simulink model "VehicleBackKin"  (R2024b)
settings: Solver=FixedStepAuto  StartTime=0.0  StopTime=inf  FixedStep=VehicleEnv.Ts  RelTol=1e-3
values from neighbouring files (symbols this model uses):
  em = ElectricMotor    [VehicleBackKinEnv.m]
  ess = VehicleEnv.ess    [VehicleBackKinEnv.m]
  fd = FinalDrive    [VehicleBackKinEnv.m]
  gb = Gearbox    [VehicleBackKinEnv.m]
  ice = Engine    [VehicleBackKinEnv.m]
  reward = VehicleEnv.reward    [VehicleBackKinEnv.m]
  selector_in = zeros(size(obs_info.Name))    [VehicleBackKinEnv.m]
  veh = Vehicle    [VehicleBackKinEnv.m]
  VehicleEnv = evalin("base","VehicleEnv")    [VehicleBackKinEnv.m]
  wh = Wheels    [VehicleBackKinEnv.m]
undefined symbols (not defined in the file or in its folder): agentSampleTime, cycle_insimulink, cycleTime, transfer_fun_coeff
libraries: simulink x3, rllib x1, autolibsharedcoreengin x1
(part 3 of 4)

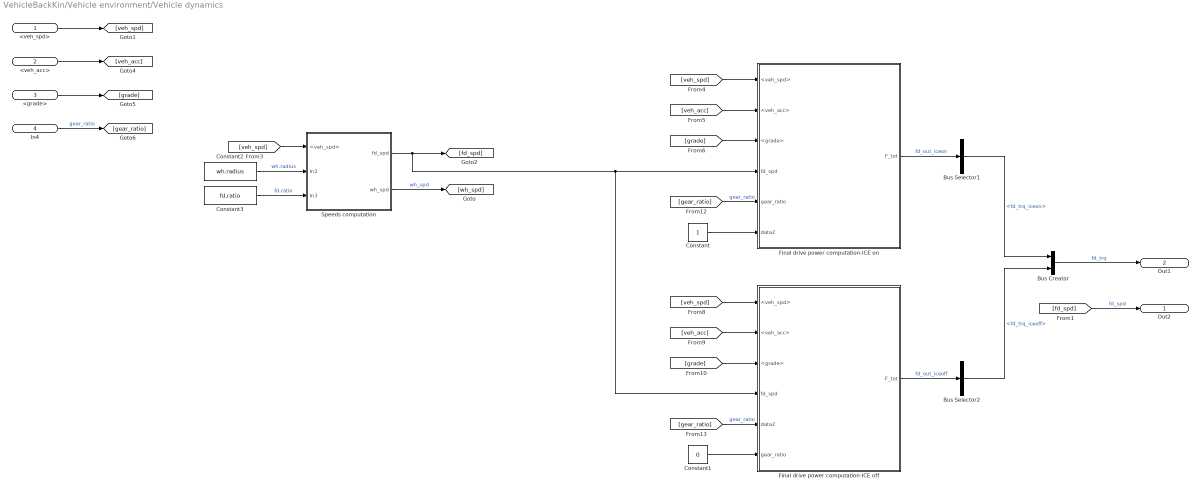
== system VehicleBackKin/Vehicle environment/Vehicle dynamics ==
  <veh_spd> : Inport
  <veh_acc> : Inport  Port=2
  <grade> : Inport  Port=3
  In4 : Inport  Port=4
  Bus Creator : BusCreator  Inputs=2
  Bus Selector1 : BusSelector  OutputSignals=fd_trq_iceon
  Bus Selector2 : BusSelector  OutputSignals=fd_trq_iceoff
  Constant : Constant
  Constant1 : Constant  Value=0
  Constant2 : Constant  Value=wh.radius
  Constant3 : Constant  Value=fd.ratio
  Final drive power computation-ICE off : Subsystem
  Final drive power computation-ICE on : Subsystem
  Speeds computation : Subsystem
  Out2 : Outport
  Out1 : Outport  Port=2
  wires:
  Speeds computation/1(fd_spd) -> [fd_spd], Final drive power computation-ICE off/4(fd_spd), Final drive power computation-ICE on/4(fd_spd)
  Speeds computation/2(wh_spd) -> [wh_spd]  "wh_spd"
  [fd_spd] -> Out2/1  "fd_spd"
  [gear_ratio] -> Final drive power computation-ICE on/5(gear_ratio)  "gear_ratio"
  <veh_spd>/1 -> [veh_spd]
  <veh_acc>/1 -> [veh_acc]
  <grade>/1 -> [grade]
  [veh_spd] -> Speeds computation/1(<veh_spd>)
  [veh_spd] -> Final drive power computation-ICE on/1(<veh_spd>)
  [veh_acc] -> Final drive power computation-ICE on/2(<veh_acc>)
  [grade] -> Final drive power computation-ICE on/3(<grade>)
  Constant/1 -> Final drive power computation-ICE on/6(data2)
  Constant1/1 -> Final drive power computation-ICE off/6(gear_ratio)
  [grade] -> Final drive power computation-ICE off/3(<grade>)
  [veh_spd] -> Final drive power computation-ICE off/1(<veh_spd>)
  [gear_ratio] -> Final drive power computation-ICE off/5(data2)  "gear_ratio"
  [veh_acc] -> Final drive power computation-ICE off/2(<veh_acc>)
  In4/1 -> [gear_ratio]  "gear_ratio"
  Constant2/1 -> Speeds computation/2(In2)  "wh.radius"
  Constant3/1 -> Speeds computation/3(In3)  "fd.ratio"
  Final drive power computation-ICE on/1(F_tot) -> Bus Selector1/1  "fd_out_iceon"
  Final drive power computation-ICE off/1(F_tot) -> Bus Selector2/1  "fd_out_iceoff"
  Bus Creator/1 -> Out1/1  "fd_trq"
  Bus Selector1/1 -> Bus Creator/1  "<fd_trq_iceon>"
  Bus Selector2/1 -> Bus Creator/2  "<fd_trq_iceoff>"

== system VehicleBackKin/Workspace saving/Testing ==
  In1 : Inport
  Bus Selector : BusSelector  OutputSignals=ice_out,batt_out,em_out,gb_out,veh_out,ems_out
  To Workspace1 : ToWorkspace  VariableName=ems_out  SaveFormat=Timeseries  SampleTime=-1
  To Workspace4 : ToWorkspace  VariableName=veh_out  SaveFormat=Timeseries  SampleTime=-1
  To Workspace5 : ToWorkspace  VariableName=gb_out  SaveFormat=Timeseries  SampleTime=-1
  To Workspace6 : ToWorkspace  VariableName=em_out  SaveFormat=Timeseries  SampleTime=-1
  To Workspace7 : ToWorkspace  VariableName=batt_out  SaveFormat=Timeseries  SampleTime=-1
  To Workspace8 : ToWorkspace  VariableName=ice_out  SaveFormat=Timeseries  SampleTime=-1
  wires:
  In1/1 -> Bus Selector/1
  Bus Selector/1 -> To Workspace8/1  "<ice_out>"
  Bus Selector/2 -> To Workspace7/1  "<batt_out>"
  Bus Selector/3 -> To Workspace6/1  "<em_out>"
  Bus Selector/4 -> To Workspace5/1  "<gb_out>"
  Bus Selector/5 -> To Workspace4/1  "<veh_out>"
  Bus Selector/6 -> To Workspace1/1  "<ems_out>"

== system VehicleBackKin/Workspace saving/Training ==
  In1 : Inport
  Bus Selector : BusSelector  OutputSignals=ice_out.ice_fuel_cum,batt_out.batt_soc
  To Workspace : ToWorkspace  VariableName=ice_fuel_cum  SaveFormat=Timeseries  SampleTime=1
  To Workspace1 : ToWorkspace  VariableName=batt_soc  SaveFormat=Timeseries  SampleTime=1
  wires:
  In1/1 -> Bus Selector/1
  Bus Selector/1 -> To Workspace/1  "<ice_fuel_cum>"
  Bus Selector/2 -> To Workspace1/1  "<batt_soc>"

== system VehicleBackKin/Reinforcement Learning controller/Reward/Dense ==
  note: Fuel penalty
  note: SoC penalty
  ice_fuel_rate : Inport
  agent_sample_time : Inport  Port=2
  batt_soc : Inport  Port=3
  Add : Sum  Inputs=+++
  Constant : Constant  Value=reward.soc_trg
  Constant1 : Constant  Value=reward.k1
  Gain : Gain  Gain=reward.k3
  Gain1 : Gain  Gain=reward.k2
  Product : Product
  SOC_reward_gain : Gain  Gain=reward.soc_gain
  Square : Math  Operator=square
  Subtract : Sum  Inputs=+-
  reward : Outport
  wires:
  Product/1 -> Gain1/1
  ice_fuel_rate/1 -> Product/1  "ice_fuel_rate"
  Add/1 -> reward/1  "reward"
  agent_sample_time/1 -> Product/2  "agent_sampleTime"
  Gain1/1 -> Add/2
  Constant1/1 -> Add/1
  Subtract/1 -> Square/1
  Constant/1 -> Subtract/2
  Gain/1 -> Add/3
  batt_soc/1 -> Subtract/1  "batt_soc"
  SOC_reward_gain/1 -> Gain/1
  Square/1 -> SOC_reward_gain/1

== system VehicleBackKin/Reinforcement Learning controller/Reward/Dense_multicycle ==
  note: Fuel penalty
  note: Distance percentage weigthing factor
  note: SoC penalty
  ice_fuel_rate : Inport
  agent_sample_time : Inport  Port=2
  batt_soc : Inport  Port=3
  veh_dist_tot : Inport  Port=4
  veh_dist_perc : Inport  Port=5
  Add : Sum  Inputs=+++
  Add1 : Sum
  Constant : Constant  Value=reward.soc_trg
  Constant1 : Constant  Value=reward.k1
  Divide : Product  Inputs=**/
  Divide1 : Product  Inputs=/*
  Gain : Gain  Gain=reward.k3*10
  Gain1 : Gain  Gain=reward.k2*10
  Gain2 : Gain  Gain=1/1000
  Product : Product
  Product1 : Product
  SOC_reward_gain : Gain  Gain=reward.soc_gain
  Square : Math  Operator=square
  Square1 : Math  Operator=square
  Subtract : Sum  Inputs=+-
  Subtract1 : Sum  Inputs=+-
  final_value : Constant
  initial_value : Constant  Value=0.3
  reward : Outport
  wires:
  Divide/1 -> Gain1/1
  ice_fuel_rate/1 -> Divide/1  "ice_fuel_rate"
  Add/1 -> reward/1  "reward"
  agent_sample_time/1 -> Divide/2  "agent_sampleTime"
  Gain1/1 -> Add/2
  Constant1/1 -> Add/1
  Constant/1 -> Subtract/2
  Gain/1 -> Add/3
  batt_soc/1 -> Subtract/1  "batt_soc"
  SOC_reward_gain/1 -> Gain/1
  veh_dist_tot/1 -> Gain2/1  "veh_dist_tot"
  Gain2/1 -> Divide1/1, Divide/3
  Subtract/1 -> Square/1
  Divide1/1 -> SOC_reward_gain/1
  Square/1 -> Product/1
  Product/1 -> Divide1/2
  Add1/1 -> Square1/1
  veh_dist_perc/1 -> Product1/1  "veh_dist_perc"
  Subtract1/1 -> Product1/2
  final_value/1 -> Subtract1/1
  Product1/1 -> Add1/1
  initial_value/1 -> Add1/2, Subtract1/2
  Square1/1 -> Product/2

== system VehicleBackKin/Reinforcement Learning controller/Reward/ECMS ==
  note: Fuel penalty
  note: Electric consumption penalty
  ice_fuel_rate : Inport
  batt_pwr : Inport  Port=2
  agent_sample_time : Inport  Port=3
  Add : Sum  Inputs=+++
  Constant1 : Constant  Value=reward.k1
  Equivalent fuel consumption : Subsystem
  Gain1 : Gain  Gain=reward.k2
  Product : Product
  reward : Outport
  wires:
  ice_fuel_rate/1 -> Product/1  "ice_fuel_rate"
  agent_sample_time/1 -> [Ts], Product/2  "agent_sampleTime"
  Product/1 -> Gain1/1
  Add/1 -> reward/1  "reward"
  Gain1/1 -> Add/2
  Constant1/1 -> Add/1
  batt_pwr/1 -> Equivalent fuel consumption/1(batt_pwr)  "batt_pwr"
  [Ts] -> Equivalent fuel consumption/2(In2)
  Equivalent fuel consumption/1(Out1) -> Add/3

== system VehicleBackKin/Reinforcement Learning controller/Reward/SOC_BC ==
  note: Fuel penalty
  note: SoC penalty
  ice_fuel_rate : Inport
  agent_sample_time : Inport  Port=2
  batt_soc : Inport  Port=3
  Add : Sum  Inputs=+++
  Constant1 : Constant  Value=reward.k1
  Gain1 : Gain  Gain=reward.k2
  Product : Product
  SoC boundary electric penalty : Subsystem
  reward : Outport
  wires:
  Constant1/1 -> Add/1
  Gain1/1 -> Add/2
  agent_sample_time/1 -> Product/2  "agent_sampleTime"
  Add/1 -> reward/1  "reward"
  ice_fuel_rate/1 -> Product/1  "ice_fuel_rate"
  Product/1 -> Gain1/1
  SoC boundary electric penalty/1(Out1) -> Add/3
  batt_soc/1 -> SoC boundary electric penalty/1(Input1)  "batt_soc"

== system VehicleBackKin/Reinforcement Learning controller/Reward/Sparse ==
  note: Fuel penalty
  note: Fuel penalty
  ice_fuel_rate : Inport
  batt_soc : Inport  Port=2
  is_done : Inport  Port=3
  agent_sample_time : Inport  Port=4
  Add : Sum  Inputs=+++
  Constant1 : Constant  Value=reward.k1
  Gain1 : Gain  Gain=reward.k2
  Product : Product
  SoC penalty : Subsystem  TreatAsAtomicUnit=on
  reward : Outport
  wires:
  SoC penalty/1(batt_soc_penalty) -> Add/2
  Add/1 -> reward/1
  is_done/1 -> SoC penalty/Enable  "is_done"
  agent_sample_time/1 -> Product/2  "agent_sampleTime"
  Product/1 -> Gain1/1
  ice_fuel_rate/1 -> Product/1  "ice_fuel_rate"
  Gain1/1 -> Add/3
  Constant1/1 -> Add/1
  batt_soc/1 -> SoC penalty/1(batt_soc)  "batt_soc"

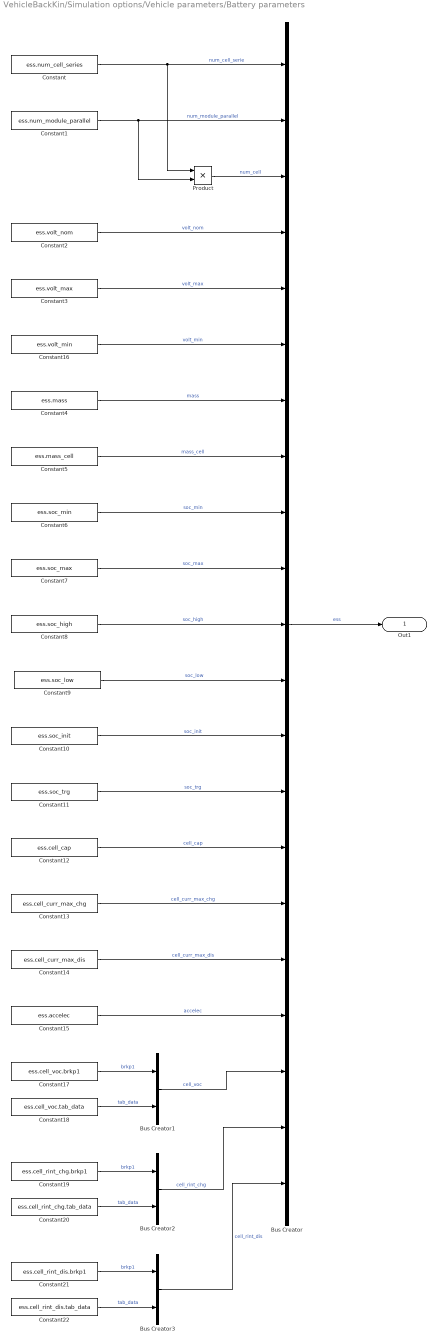
== system VehicleBackKin/Simulation options/Vehicle parameters/Battery parameters ==
  Bus Creator : BusCreator  Inputs=21
  Bus Creator1 : BusCreator  Inputs=2
  Bus Creator2 : BusCreator  Inputs=2
  Bus Creator3 : BusCreator  Inputs=2
  Constant : Constant  Value=ess.num_cell_series
  Constant1 : Constant  Value=ess.num_module_parallel
  Constant10 : Constant  Value=ess.soc_init
  Constant11 : Constant  Value=ess.soc_trg
  Constant12 : Constant  Value=ess.cell_cap
  Constant13 : Constant  Value=ess.cell_curr_max_chg
  Constant14 : Constant  Value=ess.cell_curr_max_dis
  Constant15 : Constant  Value=ess.accelec
  Constant16 : Constant  Value=ess.volt_min
  Constant17 : Constant  Value=ess.cell_voc.brkp1  VectorParams1D=off
  Constant18 : Constant  Value=ess.cell_voc.tab_data  VectorParams1D=off
  Constant19 : Constant  Value=ess.cell_rint_chg.brkp1  VectorParams1D=off
  Constant2 : Constant  Value=ess.volt_nom
  Constant20 : Constant  Value=ess.cell_rint_chg.tab_data  VectorParams1D=off
  Constant21 : Constant  Value=ess.cell_rint_dis.brkp1  VectorParams1D=off
  Constant22 : Constant  Value=ess.cell_rint_dis.tab_data  VectorParams1D=off
  Constant3 : Constant  Value=ess.volt_max
  Constant4 : Constant  Value=ess.mass
  Constant5 : Constant  Value=ess.mass_cell
  Constant6 : Constant  Value=ess.soc_min
  Constant7 : Constant  Value=ess.soc_max
  Constant8 : Constant  Value=ess.soc_high
  Constant9 : Constant  Value=ess.soc_low
  Product : Product
  Out1 : Outport
  wires:
  Constant/1 -> Bus Creator/1, Product/1  "num_cell_serie"
  Product/1 -> Bus Creator/3  "num_cell"
  Constant1/1 -> Bus Creator/2, Product/2  "num_module_parallel"
  Bus Creator/1 -> Out1/1  "ess"
  Constant2/1 -> Bus Creator/4  "volt_nom"
  Constant3/1 -> Bus Creator/5  "volt_max"
  Constant4/1 -> Bus Creator/7  "mass"
  Constant5/1 -> Bus Creator/8  "mass_cell"
  Constant6/1 -> Bus Creator/9  "soc_min"
  Constant7/1 -> Bus Creator/10  "soc_max"
  Constant8/1 -> Bus Creator/11  "soc_high"
  Constant14/1 -> Bus Creator/17  "cell_curr_max_dis"
  Constant15/1 -> Bus Creator/18  "accelec"
  Constant9/1 -> Bus Creator/12  "soc_low"
  Constant10/1 -> Bus Creator/13  "soc_init"
  Constant11/1 -> Bus Creator/14  "soc_trg"
  Constant12/1 -> Bus Creator/15  "cell_cap"
  Constant13/1 -> Bus Creator/16  "cell_curr_max_chg"
  Constant16/1 -> Bus Creator/6  "volt_min"
  Constant18/1 -> Bus Creator1/2  "tab_data"
  Constant17/1 -> Bus Creator1/1  "brkp1"
  Bus Creator1/1 -> Bus Creator/19  "cell_voc"
  Constant20/1 -> Bus Creator2/2  "tab_data"
  Constant19/1 -> Bus Creator2/1  "brkp1"
  Bus Creator2/1 -> Bus Creator/20  "cell_rint_chg"
  Constant22/1 -> Bus Creator3/2  "tab_data"
  Constant21/1 -> Bus Creator3/1  "brkp1"
  Bus Creator3/1 -> Bus Creator/21  "cell_rint_dis"

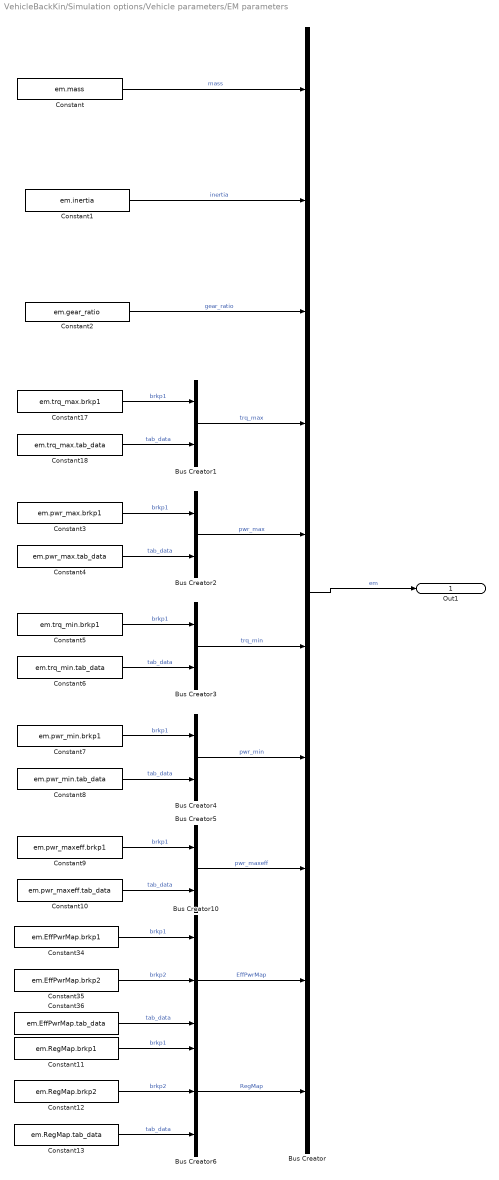
== system VehicleBackKin/Simulation options/Vehicle parameters/EM parameters ==
  Bus Creator : BusCreator  Inputs=10
  Bus Creator{1..5} (5 alike) : BusCreator  Inputs=2
  Bus Creator10 : BusCreator  Inputs=3
  Bus Creator6 : BusCreator  Inputs=3
  Constant : Constant  Value=em.mass
  Constant1 : Constant  Value=em.inertia
  Constant10 : Constant  Value=em.pwr_maxeff.tab_data  VectorParams1D=off
  Constant11 : Constant  Value=em.RegMap.brkp1  VectorParams1D=off
  Constant12 : Constant  Value=em.RegMap.brkp2  VectorParams1D=off
  Constant13 : Constant  Value=em.RegMap.tab_data  VectorParams1D=off
  Constant17 : Constant  Value=em.trq_max.brkp1  VectorParams1D=off
  Constant18 : Constant  Value=em.trq_max.tab_data  VectorParams1D=off
  Constant2 : Constant  Value=em.gear_ratio
  Constant3 : Constant  Value=em.pwr_max.brkp1  VectorParams1D=off
  Constant34 : Constant  Value=em.EffPwrMap.brkp1  VectorParams1D=off
  Constant35 : Constant  Value=em.EffPwrMap.brkp2  VectorParams1D=off
  Constant36 : Constant  Value=em.EffPwrMap.tab_data  VectorParams1D=off
  Constant4 : Constant  Value=em.pwr_max.tab_data  VectorParams1D=off
  Constant5 : Constant  Value=em.trq_min.brkp1  VectorParams1D=off
  Constant6 : Constant  Value=em.trq_min.tab_data  VectorParams1D=off
  Constant7 : Constant  Value=em.pwr_min.brkp1  VectorParams1D=off
  Constant8 : Constant  Value=em.pwr_min.tab_data  VectorParams1D=off
  Constant9 : Constant  Value=em.pwr_maxeff.brkp1  VectorParams1D=off
  Out1 : Outport
  wires:
  Bus Creator/1 -> Out1/1  "em"
  Constant1/1 -> Bus Creator/2  "inertia"
  Constant2/1 -> Bus Creator/3  "gear_ratio"
  Constant/1 -> Bus Creator/1  "mass"
  Constant17/1 -> Bus Creator1/1  "brkp1"
  Constant18/1 -> Bus Creator1/2  "tab_data"
  Bus Creator1/1 -> Bus Creator/4  "trq_max"
  Bus Creator2/1 -> Bus Creator/5  "pwr_max"
  Constant4/1 -> Bus Creator2/2  "tab_data"
  Constant3/1 -> Bus Creator2/1  "brkp1"
  Bus Creator3/1 -> Bus Creator/6  "trq_min"
  Constant6/1 -> Bus Creator3/2  "tab_data"
  Constant5/1 -> Bus Creator3/1  "brkp1"
  Bus Creator4/1 -> Bus Creator/7  "pwr_min"
  Constant8/1 -> Bus Creator4/2  "tab_data"
  Constant7/1 -> Bus Creator4/1  "brkp1"
  Bus Creator5/1 -> Bus Creator/8  "pwr_maxeff"
  Constant10/1 -> Bus Creator5/2  "tab_data"
  Constant9/1 -> Bus Creator5/1  "brkp1"
  Constant34/1 -> Bus Creator10/1  "brkp1"
  Constant35/1 -> Bus Creator10/2  "brkp2"
  Constant36/1 -> Bus Creator10/3  "tab_data"
  Bus Creator10/1 -> Bus Creator/9  "EffPwrMap"
  Bus Creator6/1 -> Bus Creator/10  "RegMap"
  Constant13/1 -> Bus Creator6/3  "tab_data"
  Constant12/1 -> Bus Creator6/2  "brkp2"
  Constant11/1 -> Bus Creator6/1  "brkp1"

== system VehicleBackKin/Simulation options/Vehicle parameters/Final drive parameters ==
  Bus Creator : BusCreator  Inputs=3
  Constant : Constant  Value=fd.ratio
  Constant1 : Constant  Value=fd.eff_max
  Constant2 : Constant  Value=fd.inertia
  Out1 : Outport
  wires:
  Constant2/1 -> Bus Creator/3  "inertia"
  Constant/1 -> Bus Creator/1  "ratio"
  Constant1/1 -> Bus Creator/2  "eff_max"
  Bus Creator/1 -> Out1/1  "fd"

== system VehicleBackKin/Simulation options/Vehicle parameters/Gearbox parameters ==
  Bus Creator : BusCreator  Inputs=6
  Constant : Constant  Value=gb.inertia_in
  Constant1 : Constant  Value=gb.inertia_out
  Constant2 : Constant  Value=gb.gear_idx
  Constant3 : Constant  Value=gb.gear_ratio
  EffTrqInMap : Subsystem
  EffTrqOutMap1 : Subsystem
  Out1 : Outport
  wires:
  Constant/1 -> Bus Creator/1  "inertia_in"
  Constant2/1 -> Bus Creator/3  "gear_idx"
  Constant1/1 -> Bus Creator/2  "inertia_out"
  Bus Creator/1 -> Out1/1  "gb"
  Constant3/1 -> Bus Creator/4  "gear_ratio"
  EffTrqInMap/1(Out1) -> Bus Creator/5
  EffTrqOutMap1/1(Out1) -> Bus Creator/6

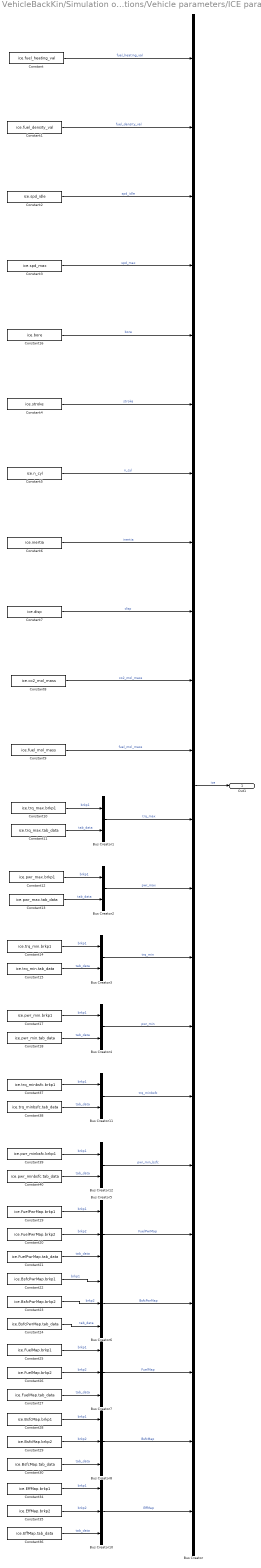
== system VehicleBackKin/Simulation options/Vehicle parameters/ICE parameters ==
  Bus Creator : BusCreator  Inputs=22
  Bus Creator{1..4,11..12} (6 alike) : BusCreator  Inputs=2
  Bus Creator{5..8,10} (5 alike) : BusCreator  Inputs=3
  Constant : Constant  Value=ice.fuel_heating_val
  Constant1 : Constant  Value=ice.fuel_density_val
  Constant10 : Constant  Value=ice.trq_max.brkp1  VectorParams1D=off
  Constant11 : Constant  Value=ice.trq_max.tab_data  VectorParams1D=off
  Constant12 : Constant  Value=ice.pwr_max.brkp1  VectorParams1D=off
  Constant13 : Constant  Value=ice.pwr_max.tab_data  VectorParams1D=off
  Constant14 : Constant  Value=ice.trq_min.brkp1  VectorParams1D=off
  Constant15 : Constant  Value=ice.trq_min.tab_data  VectorParams1D=off
  Constant16 : Constant  Value=ice.bore
  Constant17 : Constant  Value=ice.pwr_min.brkp1  VectorParams1D=off
  Constant18 : Constant  Value=ice.pwr_min.tab_data  VectorParams1D=off
  Constant19 : Constant  Value=ice.FuelPwrMap.brkp1  VectorParams1D=off
  Constant2 : Constant  Value=ice.spd_idle
  Constant20 : Constant  Value=ice.FuelPwrMap.brkp2  VectorParams1D=off
  Constant21 : Constant  Value=ice.FuelPwrMap.tab_data  VectorParams1D=off
  Constant22 : Constant  Value=ice.BsfcPwrMap.brkp1  VectorParams1D=off
  Constant23 : Constant  Value=ice.BsfcPwrMap.brkp2  VectorParams1D=off
  Constant24 : Constant  Value=ice.BsfcPwrMap.tab_data  VectorParams1D=off
  Constant25 : Constant  Value=ice.FuelMap.brkp1  VectorParams1D=off
  Constant26 : Constant  Value=ice.FuelMap.brkp2  VectorParams1D=off
  Constant27 : Constant  Value=ice.FuelMap.tab_data  VectorParams1D=off
  Constant28 : Constant  Value=ice.BsfcMap.brkp1  VectorParams1D=off
  Constant29 : Constant  Value=ice.BsfcMap.brkp2  VectorParams1D=off
  Constant3 : Constant  Value=ice.spd_max
  Constant30 : Constant  Value=ice.BsfcMap.tab_data  VectorParams1D=off
  Constant34 : Constant  Value=ice.EffMap.brkp1  VectorParams1D=off
  Constant35 : Constant  Value=ice.EffMap.brkp2  VectorParams1D=off
  Constant36 : Constant  Value=ice.EffMap.tab_data  VectorParams1D=off
  Constant37 : Constant  Value=ice.trq_minbsfc.brkp1  VectorParams1D=off
  Constant38 : Constant  Value=ice.trq_minbsfc.tab_data  VectorParams1D=off
  Constant39 : Constant  Value=ice.pwr_minbsfc.brkp1  VectorParams1D=off
  Constant4 : Constant  Value=ice.stroke
  Constant40 : Constant  Value=ice.pwr_minbsfc.tab_data  VectorParams1D=off
  Constant5 : Constant  Value=ice.n_cyl
  Constant6 : Constant  Value=ice.inertia
  Constant7 : Constant  Value=ice.disp
  Constant8 : Constant  Value=ice.co2_mol_mass
  Constant9 : Constant  Value=ice.fuel_mol_mass
  Out1 : Outport
  wires:
  Bus Creator/1 -> Out1/1  "ice"
  Constant1/1 -> Bus Creator/2  "fuel_density_val"
  Constant/1 -> Bus Creator/1  "fuel_heating_val"
  Constant2/1 -> Bus Creator/3  "spd_idle"
  Constant3/1 -> Bus Creator/4  "spd_max"
  Constant16/1 -> Bus Creator/5  "bore"
  Constant4/1 -> Bus Creator/6  "stroke"
  Constant5/1 -> Bus Creator/7  "n_cyl"
  Constant6/1 -> Bus Creator/8  "inertia"
  Constant7/1 -> Bus Creator/9  "disp"
  Constant8/1 -> Bus Creator/10  "co2_mol_mass"
  Constant9/1 -> Bus Creator/11  "fuel_mol_mass"
  Constant10/1 -> Bus Creator1/1  "brkp1"
  Constant11/1 -> Bus Creator1/2  "tab_data"
  Bus Creator1/1 -> Bus Creator/12  "trq_max"
  Bus Creator2/1 -> Bus Creator/13  "pwr_max"
  Constant13/1 -> Bus Creator2/2  "tab_data"
  Constant12/1 -> Bus Creator2/1  "brkp1"
  Constant14/1 -> Bus Creator3/1  "brkp1"
  Constant15/1 -> Bus Creator3/2  "tab_data"
  Constant18/1 -> Bus Creator4/2  "tab_data"
  Constant17/1 -> Bus Creator4/1  "brkp1"
  Constant19/1 -> Bus Creator5/1  "brkp1"
  Constant20/1 -> Bus Creator5/2  "brkp2"
  Constant21/1 -> Bus Creator5/3  "tab_data"
  Constant24/1 -> Bus Creator6/3  "tab_data"
  Constant23/1 -> Bus Creator6/2  "brkp2"
  Constant22/1 -> Bus Creator6/1  "brkp1"
  Constant25/1 -> Bus Creator7/1  "brkp1"
  Constant26/1 -> Bus Creator7/2  "brkp2"
  Constant27/1 -> Bus Creator7/3  "tab_data"
  Constant30/1 -> Bus Creator8/3  "tab_data"
  Bus Creator8/1 -> Bus Creator/21  "BsfcMap"
  Constant29/1 -> Bus Creator8/2  "brkp2"
  Constant28/1 -> Bus Creator8/1  "brkp1"
  Constant36/1 -> Bus Creator10/3  "tab_data"
  Bus Creator10/1 -> Bus Creator/22  "EffMap"
  Constant35/1 -> Bus Creator10/2  "brkp2"
  Constant34/1 -> Bus Creator10/1  "brkp1"
  Constant37/1 -> Bus Creator11/1  "brkp1"
  Constant38/1 -> Bus Creator11/2  "tab_data"
  Constant40/1 -> Bus Creator12/2  "tab_data"
  Constant39/1 -> Bus Creator12/1  "brkp1"
  Bus Creator7/1 -> Bus Creator/20  "FuelMap"
  Bus Creator6/1 -> Bus Creator/19  "BsfcPwrMap"
  Bus Creator5/1 -> Bus Creator/18  "FuelPwrMap"
  Bus Creator12/1 -> Bus Creator/17  "pwr_min_bsfc"
  Bus Creator11/1 -> Bus Creator/16  "trq_minbsfc"
  Bus Creator4/1 -> Bus Creator/15  "pwr_min"
  Bus Creator3/1 -> Bus Creator/14  "trq_min"

== system VehicleBackKin/Simulation options/Vehicle parameters/Vehicle paramateres ==
  Bus Creator : BusCreator  Inputs=6
  F0 : Constant  Value=veh.F0
  F1 : Constant  Value=veh.F1
  F2 : Constant  Value=veh.F2
  Subtract : Sum
  axal_base : Constant  Value=veh.axal_base
  body_mass : Constant  Value=veh.body_mass
  cargo_mass : Constant  Value=veh.cargo_mass
  cg_height : Constant  Value=veh.cg_height
  veh : Outport
  wires:
  Subtract/1 -> Bus Creator/3  "mass"
  cargo_mass/1 -> Subtract/1
  F0/1 -> Bus Creator/4  "F0"
  cg_height/1 -> Bus Creator/2  "cg_height"
  body_mass/1 -> Subtract/2
  F2/1 -> Bus Creator/6  "F2"
  F1/1 -> Bus Creator/5  "F1"
  axal_base/1 -> Bus Creator/1  "axal_base"
  Bus Creator/1 -> veh/1  "veh"

== system VehicleBackKin/Simulation options/Vehicle parameters/Wheels parameters ==
  Bus Creator : BusCreator  Inputs=3
  Constant : Constant  Value=wh.radius
  Constant1 : Constant  Value=wh.inertiaR
  Constant2 : Constant  Value=wh.inertiaF
  Out1 : Outport
  wires:
  Constant1/1 -> Bus Creator/2  "inertiaR"
  Constant/1 -> Bus Creator/1  "radius"
  Constant2/1 -> Bus Creator/3  "inertiaF"
  Bus Creator/1 -> Out1/1  "wh"

== system VehicleBackKin/Vehicle environment/Battery/Cell current calculation ==
  note: Cell parameters
  note: Current
  <cell_voc>1 : Inport
  In4 : Inport  Port=2
  Divide : Product  Inputs=*/
  Gain : Gain  Gain=4
  Gain1 : Gain  Gain=2
  Product : Product
  Square : Math  Operator=square
  Square Root : Sqrt
  Subtract : Sum  Inputs=+-
  Subtract1 : Sum  Inputs=+-
  Switch : Switch  SaturateOnIntegerOverflow=off  InputSameDT=off
  cell_init_chg : Lookup_n-D  NumberOfTableDimensions=1  BreakpointsForDimension1=ess.cell_rint_chg.brkp1  Table=ess.cell_rint_chg.tab_data  InternalRulePriority=Speed  RndMeth=Simplest
  cell_rint_dis : Lookup_n-D  NumberOfTableDimensions=1  BreakpointsForDimension1=ess.cell_rint_dis.brkp1  Table=ess.cell_rint_dis.tab_data  InternalRulePriority=Speed  RndMeth=Simplest
  cell_voc : Lookup_n-D  NumberOfTableDimensions=1  BreakpointsForDimension1=ess.cell_voc.brkp1  Table=ess.cell_voc.tab_data  InternalRulePriority=Speed  RndMeth=Simplest
  Out1 : Outport
  Out2 : Outport  Port=2
  Out3 : Outport  Port=3
  wires:
  cell_init_chg/1 -> Switch/3  "battc_Rchg"
  cell_voc/1 -> Out3/1, Subtract1/1, Square/1  "battc_voc"
  cell_rint_dis/1 -> Switch/1  "battc_Rdis"
  In4/1 -> [batt_soc]  "batt_soc"
  [battc_pwr] -> Switch/2
  <cell_voc>1/1 -> [battc_pwr]
  Switch/1 -> Gain1/1, Out2/1, Gain/1  "battc_R"
  Gain/1 -> Product/1
  [battc_pwr] -> Product/2
  Square/1 -> Subtract/1
  Product/1 -> Subtract/2
  Subtract/1 -> Square Root/1
  Square Root/1 -> Subtract1/2
  Subtract1/1 -> Divide/1
  Gain1/1 -> Divide/2
  Divide/1 -> Out1/1  "battc_curr"
  [batt_soc] -> cell_voc/1
  [batt_soc] -> cell_rint_dis/1
  [batt_soc] -> cell_init_chg/1

== system VehicleBackKin/Vehicle environment/Battery/Coulomb counting method ==
  note: State of charge
  note: Battery energy rate
  In1 : Inport
  <cell_cap> : Inport  Port=2
  Ah-->As : Gain  Gain=3600
  Divide : Product  Inputs=*/
  Gain : Gain  Gain=-1
  Gain1 : Gain  Gain=ess.volt_nom*ess.num_cell/1000
  Integrator : Integrator  InitialCondition=ess.soc_init
  Integrator1 : Integrator
  Product : Product
  Out1 : Outport
  Out2 : Outport  Port=2
  wires:
  Divide/1 -> Product/1, Gain/1
  Integrator/1 -> Out1/1  "batt_soc"
  In1/1 -> Divide/1  "battc_curr"
  <cell_cap>/1 -> Product/2, Ah-->As/1
  Ah-->As/1 -> Divide/2
  Gain/1 -> Integrator/1
  Product/1 -> Gain1/1
  Gain1/1 -> Integrator1/1
  Integrator1/1 -> Out2/1  "batt_en_rate [kWh]"

== system VehicleBackKin/Vehicle environment/ECU/Final drive torque management ==
  in_action : Inport
  In2 : Inport  Port=2
  In5 : Inport  Port=3
  <fd_trq_iceon> : Inport  Port=4
  <fd_trq_iceoff> : Inport  Port=5
  ice_state : Inport  Port=6
  Constant : Constant  Value=0
  Switch : Switch  Criteria=u2 > Threshold  SaturateOnIntegerOverflow=off  InputSameDT=off
  Switch1 : Switch  Criteria=u2 > Threshold  SaturateOnIntegerOverflow=off  InputSameDT=off
  Switch2 : Switch  Criteria=u2 > Threshold  SaturateOnIntegerOverflow=off  InputSameDT=off
  ice_pwr_dmd3 : Outport
  Out2 : Outport  Port=2
  Out1 : Outport  Port=3
  wires:
  ice_state/1 -> Switch/2, Switch2/2, Switch1/2
  <fd_trq_iceon>/1 -> Switch/1
  <fd_trq_iceoff>/1 -> Switch/3
  In2/1 -> Switch1/1
  In5/1 -> Switch1/3
  Switch/1 -> ice_pwr_dmd3/1  "fd_trq"
  Switch1/1 -> Out2/1  "fd_pwr"
  in_action/1 -> Switch2/1
  Constant/1 -> Switch2/3
  Switch2/1 -> Out1/1  "action"

== system VehicleBackKin/Vehicle environment/ECU/ICE state controller ==
  In1 : Inport
  Input2 : Inport  Port=2
  Constant : Constant
  Constant1 : Constant  Value=0
  Constant2 : Constant  Value=0
  Switch : Switch  Criteria=u2 > Threshold  Threshold=0.2  SaturateOnIntegerOverflow=off  InputSameDT=off
  Switch1 : Switch  Criteria=u2 > Threshold  SaturateOnIntegerOverflow=off  InputSameDT=off
  ice_pwr_dmd2 : Outport
  wires:
  Constant/1 -> Switch/1
  Constant1/1 -> Switch/3
  Switch/1 -> Switch1/1
  Input2/1 -> Switch/2
  In1/1 -> Switch1/2
  Constant2/1 -> Switch1/3
  Switch1/1 -> ice_pwr_dmd2/1  "ice_state"

== system VehicleBackKin/Vehicle environment/ECU/Limit computation ==
  In1 : Inport
  In2 : Inport  Port=2
  1-D Lookup Table : Lookup_n-D  NumberOfTableDimensions=1  BreakpointsForDimension1=ice.pwr_max.brkp1  Table=ice.pwr_max.tab_data  InternalRulePriority=Speed  RndMeth=Simplest
  1-D Lookup Table1 : Lookup_n-D  NumberOfTableDimensions=1  BreakpointsForDimension1=ice.pwr_min.brkp1  Table=ice.pwr_min.tab_data  InternalRulePriority=Speed  RndMeth=Simplest
  1-D Lookup Table2 : Lookup_n-D  NumberOfTableDimensions=1  BreakpointsForDimension1=ice.trq_max.brkp1  Table=ice.trq_max.tab_data  InternalRulePriority=Speed  RndMeth=Simplest
  1-D Lookup Table3 : Lookup_n-D  NumberOfTableDimensions=1  BreakpointsForDimension1=em.pwr_max.brkp1  Table=em.pwr_max.tab_data  InternalRulePriority=Speed  RndMeth=Simplest
  1-D Lookup Table4 : Lookup_n-D  NumberOfTableDimensions=1  BreakpointsForDimension1=em.pwr_min.brkp1  Table=em.pwr_min.tab_data  InternalRulePriority=Speed  RndMeth=Simplest
  ice_max_pwr : Outport
  ice_min_pwr : Outport  Port=2
  ice_max_trq : Outport  Port=3
  ice_max_pwr1 : Outport  Port=4
  ice_min_pwr1 : Outport  Port=5
  wires:
  In2/1 -> 1-D Lookup Table3/1, 1-D Lookup Table4/1
  1-D Lookup Table3/1 -> ice_max_pwr1/1  "em_pwr_max"
  In1/1 -> 1-D Lookup Table2/1, 1-D Lookup Table1/1, 1-D Lookup Table/1
  1-D Lookup Table2/1 -> ice_max_trq/1  "ice_trq_max"
  1-D Lookup Table4/1 -> ice_min_pwr1/1  "em_pwr_min"
  1-D Lookup Table/1 -> ice_max_pwr/1  "ice_pwr_max"
  1-D Lookup Table1/1 -> ice_min_pwr/1  "ice_pwr_min"

== system VehicleBackKin/Vehicle environment/ECU/Regenerative braking ==
  In1 : Inport
  In2 : Inport  Port=2
  Input : Inport  Port=3
  2-D Lookup Table : Lookup_n-D  BreakpointsForDimension1=em.RegMap.brkp2  BreakpointsForDimension2=em.RegMap.brkp1  Table=em.RegMap.tab_data  ExtrapMethod=Clip  InternalRulePriority=Speed  RndMeth=Simplest
      settings: InputPortMap=u0,u1
  Product2 : Product
  Scope : Scope
  Scope1 : Scope  NumInputPorts=2
  data2 : Outport
  wires:
  2-D Lookup Table/1 -> Scope/1, Product2/2  "reg_brk_factor"
  Product2/1 -> Scope1/2, data2/1  "em_pwr_reg"
  Input/1 -> Scope1/1, Product2/1
  In1/1 -> 2-D Lookup Table/1
  In2/1 -> 2-D Lookup Table/2

== system VehicleBackKin/Vehicle environment/ECU/Traction power demand ==
  ice_max_pwr : Inport
  ice_min_pwr : Inport  Port=2
  ice_max_trq : Inport  Port=3
  ice_max_pwr1 : Inport  Port=4
  ice_min_pwr1 : Inport  Port=5
  Input : Inport  Port=6
  In6 : Inport  Port=7
  ice_min_pwr2 : Inport  Port=8
  ice_max_trq1 : Inport  Port=9
  Constant : Constant  Value=0
  Product : Product
  Product1 : Product
  Saturation Dynamic : simulink/Discontinuities/Saturation Dynamic  OutMin=[]  OutMax=[]  OutDataTypeStr=Inherit: Same as second input  OutDataType=fixdt(1, 16)  OutScaling=2^-10  DoSatur=off
  Saturation Dynamic1 : simulink/Discontinuities/Saturation Dynamic  OutMin=[]  OutMax=[]  OutDataTypeStr=Inherit: Same as second input  OutDataType=fixdt(1, 16)  OutScaling=2^-10  DoSatur=off
  Subtract : Sum  Inputs=-+
  Switch : Switch  Criteria=u2 > Threshold  SaturateOnIntegerOverflow=off  InputSameDT=off
  ice_pwr_dmd : Outport
  Out2 : Outport  Port=2
  wires:
  Saturation Dynamic1/1 -> Out2/1  "em_pwr_trac"
  ice_min_pwr/1 -> Saturation Dynamic/3
  ice_min_pwr1/1 -> Saturation Dynamic1/3
  Product/1 -> Product1/1  "ice_trq"
  Switch/1 -> Subtract/1
  ice_max_pwr1/1 -> Saturation Dynamic1/1
  Subtract/1 -> Saturation Dynamic1/2  "em_pwr"
  ice_max_trq1/1 -> Product/1  "action"
  ice_max_pwr/1 -> Saturation Dynamic/1
  Saturation Dynamic/1 -> ice_pwr_dmd/1, Switch/1  "ice_pwr_trac"
  In6/1 -> Product1/2
  ice_min_pwr2/1 -> Switch/2
  Input/1 -> Subtract/2
  Product1/1 -> Saturation Dynamic/2  "ice_pwr"
  Constant/1 -> Switch/3
  ice_max_trq/1 -> Product/2

== system VehicleBackKin/Vehicle environment/Internal combustion engine/CO2 computation ==
  In3 : Inport
  <co2_mol_mass> : Inport  Port=2
  <fuel_mol_mass> : Inport  Port=3
  Divide : Product  Inputs=*/*
  Integrator : Integrator
  Out1 : Outport
  Out2 : Outport  Port=2
  wires:
  Divide/1 -> Integrator/1, Out1/1  "ice_co2_rate"
  In3/1 -> Divide/3
  <co2_mol_mass>/1 -> Divide/1
  <fuel_mol_mass>/1 -> Divide/2
  Integrator/1 -> Out2/1  "ice_co2_cum"

== system VehicleBackKin/Vehicle environment/Internal combustion engine/Fuel cut-off ==
  note: lessthan constant
  note: Cut-off
  In1 : Inport
  In2 : Inport  Port=2
  In3 : Inport  Port=3
  <spd_idle> : Inport  Port=4
  ice_pwr_dmd : Inport  Port=5
  AND : Logic  IconShape=distinctive  AllPortsSameDT=off  OutDataTypeStr=boolean
  Compare To Constant : simulink/Logic and Bit Operations/Compare To Constant  relop=<=  const=0  OutDataTypeStr=boolean
  Constant : Constant  Value=0
  Constant2 : Constant  Value=0  VectorParams1D=off  SampleTime=-1
  GreaterThan : RelationalOperator  Operator=>  OutDataTypeStr=boolean  RndMeth=Simplest  InputSameDT=off
  Switch : Switch  Criteria=u2 > Threshold  SaturateOnIntegerOverflow=off  InputSameDT=off
  Switch1 : Switch  Criteria=u2 > Threshold  SaturateOnIntegerOverflow=off  InputSameDT=off
  Out1 : Outport
  wires:
  <spd_idle>/1 -> GreaterThan/2
  In3/1 -> GreaterThan/1
  ice_pwr_dmd/1 -> Compare To Constant/1
  GreaterThan/1 -> AND/1
  Compare To Constant/1 -> AND/2
  Switch/1 -> Switch1/3
  AND/1 -> Switch1/2
  Switch1/1 -> Out1/1  "ice_fuel_rate"
  Constant/1 -> Switch/3
  In1/1 -> Switch/1  "ice_fuel_rate_map"
  In2/1 -> Switch/2  "ice_state"
  Constant2/1 -> Switch1/1

== system VehicleBackKin/Vehicle environment/Internal combustion engine/Speed calculation ==
  In1 : Inport
  ice_state : Inport  Port=2
  In2 : Inport  Port=3
  Constant : Constant  Value=0
  Max : MinMax  Function=max  Inputs=2
  Switch : Switch  Criteria=u2 > Threshold  SaturateOnIntegerOverflow=off  InputSameDT=off
  Out1 : Outport
  wires:
  Switch/1 -> Out1/1  "ice_spd"
  Constant/1 -> Switch/3
  In1/1 -> Max/1
  Max/1 -> Switch/1  "ice_spd"
  ice_state/1 -> Switch/2
  In2/1 -> Max/2

== system VehicleBackKin/Vehicle environment/Vehicle dynamics/Final drive power computation-ICE off ==
  <veh_spd> : Inport
  <veh_acc> : Inport  Port=2
  <grade> : Inport  Port=3
  fd_spd : Inport  Port=4
  data2 : Inport  Port=5
  gear_ratio : Inport  Port=6
  Road load power computation : Subsystem
  Vehicle equivalent mass : Subsystem
  F_tot : Outport
  wires:
  Vehicle equivalent mass/1(Out1) -> Road load power computation/5(In5)
  fd_spd/1 -> Road load power computation/4(fd_spd)
  <veh_acc>/1 -> Road load power computation/2(<veh_acc>)
  <veh_spd>/1 -> Road load power computation/1(<veh_spd>)
  gear_ratio/1 -> Vehicle equivalent mass/1(In2)
  <grade>/1 -> Road load power computation/3(<grade>)
  data2/1 -> Vehicle equivalent mass/2(data2)  "ice_state"
  Road load power computation/1(F_tot) -> F_tot/1

== system VehicleBackKin/Vehicle environment/Vehicle dynamics/Final drive power computation-ICE on ==
  <veh_spd> : Inport
  <veh_acc> : Inport  Port=2
  <grade> : Inport  Port=3
  fd_spd : Inport  Port=4
  gear_ratio : Inport  Port=5
  data2 : Inport  Port=6
  Road load power computation : Subsystem
  Vehicle equivalent mass : Subsystem
  F_tot : Outport
  wires:
  Vehicle equivalent mass/1(Out1) -> Road load power computation/5(In5)
  fd_spd/1 -> Road load power computation/4(fd_spd)
  <veh_acc>/1 -> Road load power computation/2(<veh_acc>)
  <veh_spd>/1 -> Road load power computation/1(<veh_spd>)
  gear_ratio/1 -> Vehicle equivalent mass/1(In2)
  <grade>/1 -> Road load power computation/3(<grade>)
  data2/1 -> Vehicle equivalent mass/2(data2)  "ice_state"
  Road load power computation/1(F_tot) -> F_tot/1

== system VehicleBackKin/Vehicle environment/Vehicle dynamics/Speeds computation ==
  <veh_spd> : Inport
  In2 : Inport  Port=2
  In3 : Inport  Port=3
  Divide : Product  Inputs=*/
  Product : Product
  fd_spd : Outport
  wh_spd : Outport  Port=2
  wires:
  Divide/1 -> wh_spd/1, Product/1  "wh_spd"
  <veh_spd>/1 -> Divide/1
  Product/1 -> fd_spd/1  "fd_spd"
  In3/1 -> Product/2
  In2/1 -> Divide/2

== system VehicleBackKin/Reinforcement Learning controller/Reward/ECMS/Equivalent fuel consumption ==
  batt_pwr : Inport
  In2 : Inport  Port=2
  Constant : Constant  Value=reward.eff_dis
  Constant2 : Constant  Value=reward.eff_chg
  Constant3 : Constant  Value=ice.fuel_heating_val
  Divide : Product  Inputs=*/
  Divide1 : Product  Inputs=*/
  Gain2 : Gain  Gain=reward.k3
  Product1 : Product
  Product2 : Product
  Switch : Switch  SaturateOnIntegerOverflow=off  InputSameDT=off
  Out1 : Outport
  wires:
  Product1/1 -> Switch/3
  Gain2/1 -> Divide1/1
  batt_pwr/1 -> Divide/1, Product1/1, Switch/2
  Constant/1 -> Divide/2
  In2/1 -> Product2/2  "Ts"
  Constant2/1 -> Product1/2
  Divide1/1 -> Product2/1
  Divide/1 -> Switch/1
  Constant3/1 -> Divide1/2
  Switch/1 -> Gain2/1
  Product2/1 -> Out1/1  "equivalent_fuel_consumption"

== system VehicleBackKin/Reinforcement Learning controller/Reward/SOC_BC/SoC boundary electric penalty ==
  Input1 : Inport
  Constant : Constant  Value=reward.soc_trg
  Constant1 : Constant  Value=reward.soc_trg
  Constant2 : Constant  Value=2*reward.soc_trg
  From Workspace : FromWorkspace  VariableName=reward_bc
  Gain : Gain  Gain=reward.k3
  Gain1 : Gain  Gain=reward.k3
  Gain2 : Gain  Gain=reward.soc_bc_gain
  GreaterThanOrEqual : RelationalOperator  OutDataTypeStr=boolean  RndMeth=Simplest  InputSameDT=off
  LowerThanOrEqua1 : RelationalOperator  Operator=<=  OutDataTypeStr=boolean  RndMeth=Simplest  InputSameDT=off
  OR : Logic  Operator=OR  IconShape=distinctive  AllPortsSameDT=off  OutDataTypeStr=boolean
  SOC_reward_gain : Gain  Gain=reward.soc_gain
  SOC_reward_gain1 : Gain  Gain=reward.soc_gain
  Square : Math  Operator=square
  Square1 : Math  Operator=square
  Subtract : Sum  Inputs=+-
  Subtract1 : Sum  Inputs=+-
  Subtract2 : Sum  Inputs=-+
  Switch : Switch  Criteria=u2 > Threshold  SaturateOnIntegerOverflow=off  InputSameDT=off
  Out1 : Outport
  wires:
  From Workspace/1 -> Subtract2/1, GreaterThanOrEqual/2  "soc_bc_up"
  Gain1/1 -> Gain2/1
  Subtract2/1 -> LowerThanOrEqua1/2  "soc_bc_low"
  OR/1 -> Switch/2
  Constant2/1 -> Subtract2/2
  GreaterThanOrEqual/1 -> OR/1
  Gain/1 -> Switch/1
  LowerThanOrEqua1/1 -> OR/2
  [batt_soc] -> LowerThanOrEqua1/1
  Switch/1 -> Out1/1  "batt_soc_penalty"
  Input1/1 -> [batt_soc]
  Constant/1 -> Subtract/2
  Square/1 -> SOC_reward_gain/1
  SOC_reward_gain/1 -> Gain/1
  [batt_soc] -> Subtract/1  "batt_soc"
  Subtract/1 -> Square/1
  [batt_soc] -> GreaterThanOrEqual/1
  SOC_reward_gain1/1 -> Gain1/1
  Subtract1/1 -> Square1/1
  Constant1/1 -> Subtract1/2
  [batt_soc] -> Subtract1/1  "batt_soc"
  Square1/1 -> SOC_reward_gain1/1
  Gain2/1 -> Switch/3

== system VehicleBackKin/Reinforcement Learning controller/Reward/Sparse/SoC penalty ==
  batt_soc : Inport
  Enable : EnablePort  StatesWhenEnabling=reset
  Constant3 : Constant  Value=reward.soc_trg
  Gain : Gain  Gain=reward.k3
  SOC_reward_gain : Gain  Gain=reward.soc_gain
  Square : Math  Operator=square
  Subtract1 : Sum  Inputs=+-
  batt_soc_penalty : Outport
  wires:
  Constant3/1 -> Subtract1/2
  Subtract1/1 -> Square/1
  batt_soc/1 -> Subtract1/1  "batt_soc"
  SOC_reward_gain/1 -> Gain/1
  Square/1 -> SOC_reward_gain/1
  Gain/1 -> batt_soc_penalty/1  "batt_soc_penalty"

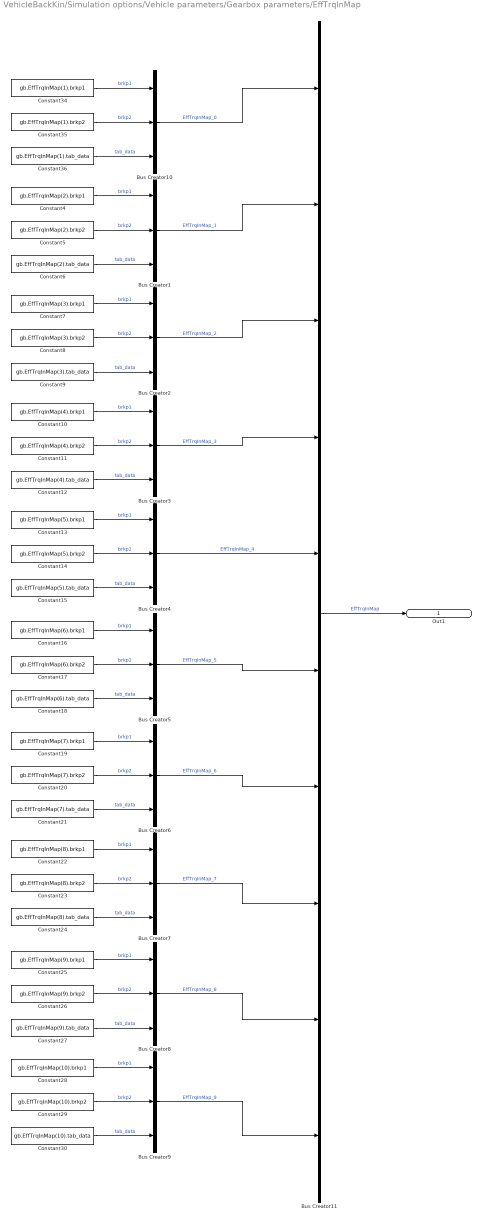
== system VehicleBackKin/Simulation options/Vehicle parameters/Gearbox parameters/EffTrqInMap ==
  Bus Creator{1..10} (10 alike) : BusCreator  Inputs=3
  Bus Creator11 : BusCreator  Inputs=10
  Constant10 : Constant  Value=gb.EffTrqInMap(4).brkp1
  Constant11 : Constant  Value=gb.EffTrqInMap(4).brkp2
  Constant12 : Constant  Value=gb.EffTrqInMap(4).tab_data
  Constant13 : Constant  Value=gb.EffTrqInMap(5).brkp1
  Constant14 : Constant  Value=gb.EffTrqInMap(5).brkp2
  Constant15 : Constant  Value=gb.EffTrqInMap(5).tab_data
  Constant16 : Constant  Value=gb.EffTrqInMap(6).brkp1
  Constant17 : Constant  Value=gb.EffTrqInMap(6).brkp2
  Constant18 : Constant  Value=gb.EffTrqInMap(6).tab_data
  Constant19 : Constant  Value=gb.EffTrqInMap(7).brkp1
  Constant20 : Constant  Value=gb.EffTrqInMap(7).brkp2
  Constant21 : Constant  Value=gb.EffTrqInMap(7).tab_data
  Constant22 : Constant  Value=gb.EffTrqInMap(8).brkp1
  Constant23 : Constant  Value=gb.EffTrqInMap(8).brkp2
  Constant24 : Constant  Value=gb.EffTrqInMap(8).tab_data
  Constant25 : Constant  Value=gb.EffTrqInMap(9).brkp1
  Constant26 : Constant  Value=gb.EffTrqInMap(9).brkp2
  Constant27 : Constant  Value=gb.EffTrqInMap(9).tab_data
  Constant28 : Constant  Value=gb.EffTrqInMap(10).brkp1
  Constant29 : Constant  Value=gb.EffTrqInMap(10).brkp2
  Constant30 : Constant  Value=gb.EffTrqInMap(10).tab_data
  Constant34 : Constant  Value=gb.EffTrqInMap(1).brkp1
  Constant35 : Constant  Value=gb.EffTrqInMap(1).brkp2
  Constant36 : Constant  Value=gb.EffTrqInMap(1).tab_data
  Constant4 : Constant  Value=gb.EffTrqInMap(2).brkp1
  Constant5 : Constant  Value=gb.EffTrqInMap(2).brkp2
  Constant6 : Constant  Value=gb.EffTrqInMap(2).tab_data
  Constant7 : Constant  Value=gb.EffTrqInMap(3).brkp1
  Constant8 : Constant  Value=gb.EffTrqInMap(3).brkp2
  Constant9 : Constant  Value=gb.EffTrqInMap(3).tab_data
  Out1 : Outport
  wires:
  Constant18/1 -> Bus Creator5/3  "tab_data"
  Constant22/1 -> Bus Creator7/1  "brkp1"
  Bus Creator3/1 -> Bus Creator11/4  "EffTrqInMap_3"
  Constant29/1 -> Bus Creator9/2  "brkp2"
  Constant7/1 -> Bus Creator2/1  "brkp1"
  Constant5/1 -> Bus Creator1/2  "brkp2"
  Constant10/1 -> Bus Creator3/1  "brkp1"
  Constant25/1 -> Bus Creator8/1  "brkp1"
  Constant19/1 -> Bus Creator6/1  "brkp1"
  Constant35/1 -> Bus Creator10/2  "brkp2"
  Bus Creator1/1 -> Bus Creator11/2  "EffTrqInMap_1"
  Bus Creator5/1 -> Bus Creator11/6  "EffTrqInMap_5"
  Constant11/1 -> Bus Creator3/2  "brkp2"
  Constant12/1 -> Bus Creator3/3  "tab_data"
  Bus Creator8/1 -> Bus Creator11/9  "EffTrqInMap_8"
  Constant4/1 -> Bus Creator1/1  "brkp1"
  Constant17/1 -> Bus Creator5/2  "brkp2"
  Constant21/1 -> Bus Creator6/3  "tab_data"
  Bus Creator7/1 -> Bus Creator11/8  "EffTrqInMap_7"
  Constant16/1 -> Bus Creator5/1  "brkp1"
  Constant36/1 -> Bus Creator10/3  "tab_data"
  Constant24/1 -> Bus Creator7/3  "tab_data"
  Constant34/1 -> Bus Creator10/1  "brkp1"
  Constant28/1 -> Bus Creator9/1  "brkp1"
  Bus Creator10/1 -> Bus Creator11/1  "EffTrqInMap_0"
  Constant30/1 -> Bus Creator9/3  "tab_data"
  Constant23/1 -> Bus Creator7/2  "brkp2"
  Bus Creator11/1 -> Out1/1  "EffTrqInMap"
  Constant20/1 -> Bus Creator6/2  "brkp2"
  Constant26/1 -> Bus Creator8/2  "brkp2"
  Constant13/1 -> Bus Creator4/1  "brkp1"
  Constant14/1 -> Bus Creator4/2  "brkp2"
  Constant15/1 -> Bus Creator4/3  "tab_data"
  Bus Creator2/1 -> Bus Creator11/3  "EffTrqInMap_2"
  Bus Creator9/1 -> Bus Creator11/10  "EffTrqInMap_9"
  Bus Creator4/1 -> Bus Creator11/5  "EffTrqInMap_4"
  Constant9/1 -> Bus Creator2/3  "tab_data"
  Constant27/1 -> Bus Creator8/3  "tab_data"
  Constant8/1 -> Bus Creator2/2  "brkp2"
  Bus Creator6/1 -> Bus Creator11/7  "EffTrqInMap_6"
  Constant6/1 -> Bus Creator1/3  "tab_data"

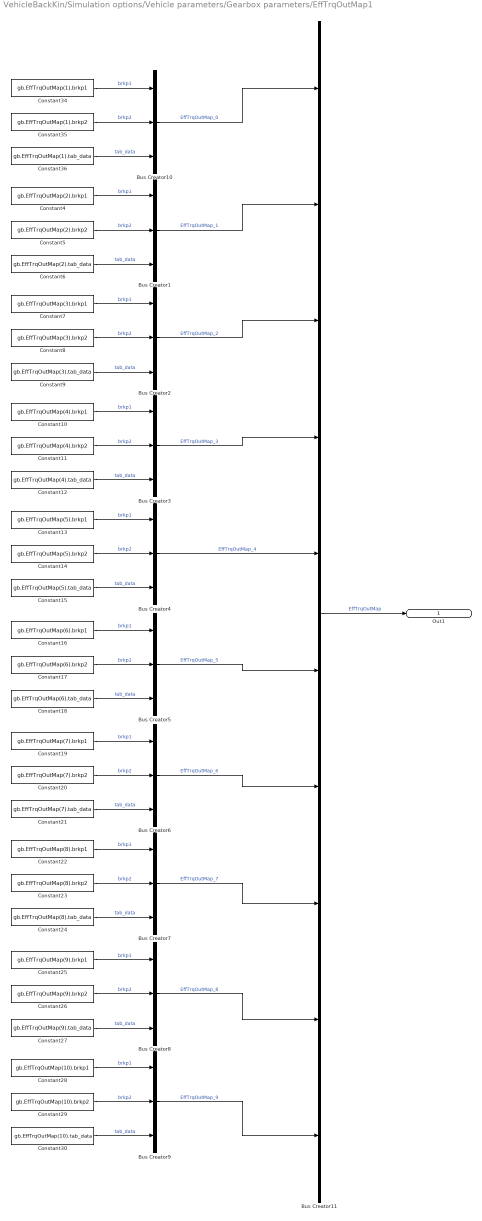
== system VehicleBackKin/Simulation options/Vehicle parameters/Gearbox parameters/EffTrqOutMap1 ==
  Bus Creator{1..10} (10 alike) : BusCreator  Inputs=3
  Bus Creator11 : BusCreator  Inputs=10
  Constant10 : Constant  Value=gb.EffTrqOutMap(4).brkp1
  Constant11 : Constant  Value=gb.EffTrqOutMap(4).brkp2
  Constant12 : Constant  Value=gb.EffTrqOutMap(4).tab_data
  Constant13 : Constant  Value=gb.EffTrqOutMap(5).brkp1
  Constant14 : Constant  Value=gb.EffTrqOutMap(5).brkp2
  Constant15 : Constant  Value=gb.EffTrqOutMap(5).tab_data
  Constant16 : Constant  Value=gb.EffTrqOutMap(6).brkp1
  Constant17 : Constant  Value=gb.EffTrqOutMap(6).brkp2
  Constant18 : Constant  Value=gb.EffTrqOutMap(6).tab_data
  Constant19 : Constant  Value=gb.EffTrqOutMap(7).brkp1
  Constant20 : Constant  Value=gb.EffTrqOutMap(7).brkp2
  Constant21 : Constant  Value=gb.EffTrqOutMap(7).tab_data
  Constant22 : Constant  Value=gb.EffTrqOutMap(8).brkp1
  Constant23 : Constant  Value=gb.EffTrqOutMap(8).brkp2
  Constant24 : Constant  Value=gb.EffTrqOutMap(8).tab_data
  Constant25 : Constant  Value=gb.EffTrqOutMap(9).brkp1
  Constant26 : Constant  Value=gb.EffTrqOutMap(9).brkp2
  Constant27 : Constant  Value=gb.EffTrqOutMap(9).tab_data
  Constant28 : Constant  Value=gb.EffTrqOutMap(10).brkp1
  Constant29 : Constant  Value=gb.EffTrqOutMap(10).brkp2
  Constant30 : Constant  Value=gb.EffTrqOutMap(10).tab_data
  Constant34 : Constant  Value=gb.EffTrqOutMap(1).brkp1
  Constant35 : Constant  Value=gb.EffTrqOutMap(1).brkp2
  Constant36 : Constant  Value=gb.EffTrqOutMap(1).tab_data
  Constant4 : Constant  Value=gb.EffTrqOutMap(2).brkp1
  Constant5 : Constant  Value=gb.EffTrqOutMap(2).brkp2
  Constant6 : Constant  Value=gb.EffTrqOutMap(2).tab_data
  Constant7 : Constant  Value=gb.EffTrqOutMap(3).brkp1
  Constant8 : Constant  Value=gb.EffTrqOutMap(3).brkp2
  Constant9 : Constant  Value=gb.EffTrqOutMap(3).tab_data
  Out1 : Outport
  wires:
  Constant18/1 -> Bus Creator5/3  "tab_data"
  Constant22/1 -> Bus Creator7/1  "brkp1"
  Bus Creator3/1 -> Bus Creator11/4  "EffTrqOutMap_3"
  Constant29/1 -> Bus Creator9/2  "brkp2"
  Constant7/1 -> Bus Creator2/1  "brkp1"
  Constant5/1 -> Bus Creator1/2  "brkp2"
  Constant10/1 -> Bus Creator3/1  "brkp1"
  Constant25/1 -> Bus Creator8/1  "brkp1"
  Constant19/1 -> Bus Creator6/1  "brkp1"
  Constant35/1 -> Bus Creator10/2  "brkp2"
  Bus Creator1/1 -> Bus Creator11/2  "EffTrqOutMap_1"
  Bus Creator5/1 -> Bus Creator11/6  "EffTrqOutMap_5"
  Constant11/1 -> Bus Creator3/2  "brkp2"
  Constant12/1 -> Bus Creator3/3  "tab_data"
  Bus Creator8/1 -> Bus Creator11/9  "EffTrqOutMap_8"
  Constant4/1 -> Bus Creator1/1  "brkp1"
  Constant17/1 -> Bus Creator5/2  "brkp2"
  Constant21/1 -> Bus Creator6/3  "tab_data"
  Bus Creator7/1 -> Bus Creator11/8  "EffTrqOutMap_7"
  Constant16/1 -> Bus Creator5/1  "brkp1"
  Constant36/1 -> Bus Creator10/3  "tab_data"
  Constant24/1 -> Bus Creator7/3  "tab_data"
  Constant34/1 -> Bus Creator10/1  "brkp1"
  Constant28/1 -> Bus Creator9/1  "brkp1"
  Bus Creator10/1 -> Bus Creator11/1  "EffTrqOutMap_0"
  Constant30/1 -> Bus Creator9/3  "tab_data"
  Constant23/1 -> Bus Creator7/2  "brkp2"
  Bus Creator11/1 -> Out1/1  "EffTrqOutMap"
  Constant20/1 -> Bus Creator6/2  "brkp2"
  Constant26/1 -> Bus Creator8/2  "brkp2"
  Constant13/1 -> Bus Creator4/1  "brkp1"
  Constant14/1 -> Bus Creator4/2  "brkp2"
  Constant15/1 -> Bus Creator4/3  "tab_data"
  Bus Creator2/1 -> Bus Creator11/3  "EffTrqOutMap_2"
  Bus Creator9/1 -> Bus Creator11/10  "EffTrqOutMap_9"
  Bus Creator4/1 -> Bus Creator11/5  "EffTrqOutMap_4"
  Constant9/1 -> Bus Creator2/3  "tab_data"
  Constant27/1 -> Bus Creator8/3  "tab_data"
  Constant8/1 -> Bus Creator2/2  "brkp2"
  Bus Creator6/1 -> Bus Creator11/7  "EffTrqOutMap_6"
  Constant6/1 -> Bus Creator1/3  "tab_data"

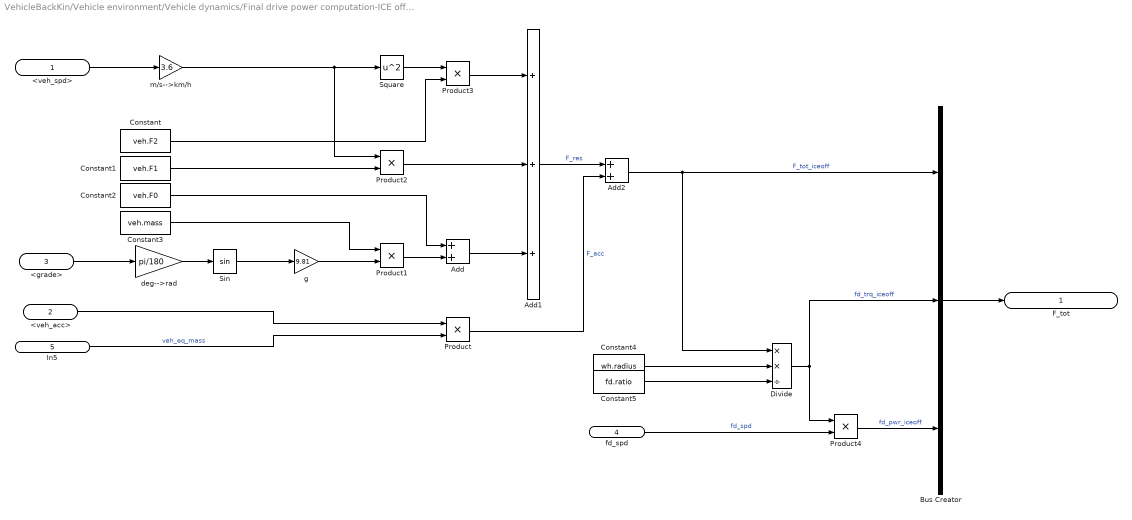
== system VehicleBackKin/Vehicle environment/Vehicle dynamics/Final drive power computation-ICE off/Road load power computation ==
  <veh_spd> : Inport
  <veh_acc> : Inport  Port=2
  <grade> : Inport  Port=3
  fd_spd : Inport  Port=4
  In5 : Inport  Port=5
  Add : Sum
  Add1 : Sum  Inputs=+++
  Add2 : Sum
  Bus Creator : BusCreator  Inputs=3
  Constant : Constant  Value=veh.F2
  Constant1 : Constant  Value=veh.F1
  Constant2 : Constant  Value=veh.F0
  Constant3 : Constant  Value=veh.mass
  Constant4 : Constant  Value=wh.radius
  Constant5 : Constant  Value=fd.ratio
  Divide : Product  Inputs=**/
  Product{,1..4} (5 alike) : Product
  Sin : Trigonometry
  Square : Math  Operator=square
  deg-->rad : Gain  Gain=pi/180
  g : Gain  Gain=9.81
  m/s-->km/h : Gain  Gain=3.6
  F_tot : Outport
  wires:
  <veh_spd>/1 -> m/s-->km/h/1
  <grade>/1 -> deg-->rad/1
  deg-->rad/1 -> Sin/1
  Constant1/1 -> Product2/2
  Sin/1 -> g/1
  m/s-->km/h/1 -> Product2/1, Square/1
  Constant2/1 -> Add/1
  Constant3/1 -> Product1/1
  g/1 -> Product1/2
  Product2/1 -> Add1/2
  Product1/1 -> Add/2
  Product3/1 -> Add1/1
  Add1/1 -> Add2/1  "F_res"
  Add/1 -> Add1/3
  <veh_acc>/1 -> Product/1
  In5/1 -> Product/2  "veh_eq_mass"
  Add2/1 -> Divide/1, Bus Creator/1  "F_tot_iceoff"
  Product/1 -> Add2/2  "F_acc"
  Constant/1 -> Product3/2
  Square/1 -> Product3/1
  Constant4/1 -> Divide/2
  Constant5/1 -> Divide/3
  Divide/1 -> Bus Creator/2, Product4/1  "fd_trq_iceoff"
  fd_spd/1 -> Product4/2  "fd_spd"
  Product4/1 -> Bus Creator/3  "fd_pwr_iceoff"
  Bus Creator/1 -> F_tot/1

== system VehicleBackKin/Vehicle environment/Vehicle dynamics/Final drive power computation-ICE off/Vehicle equivalent mass ==
  note: Wheel
  note: ICE
  note: EM
  In2 : Inport
  data2 : Inport  Port=2
  Add : Sum
  Add1 : Sum  Inputs=++++
  Constant : Constant  Value=0
  Constant2 : Constant  Value=veh.mass
  Constant3 : Constant  Value=wh.inertiaR
  Constant4 : Constant  Value=wh.inertiaF
  Constant5 : Constant  Value=wh.radius
  Constant6 : Constant  Value=ice.inertia
  Constant7 : Constant  Value=fd.ratio
  Constant8 : Constant  Value=em.inertia
  Constant9 : Constant  Value=em.gear_ratio
  Divide : Product  Inputs=*/
  Divide1 : Product  Inputs=/*
  Divide2 : Product  Inputs=/*
  Gain : Gain  Gain=2
  Product : Product
  Product1 : Product
  Product2 : Product  Inputs=3
  Square : Math  Operator=square
  Square1 : Math  Operator=square
  Square2 : Math  Operator=square
  Switch : Switch  Criteria=u2 > Threshold  SaturateOnIntegerOverflow=off  InputSameDT=off
  Out1 : Outport
  wires:
  Constant3/1 -> Add/1
  Square1/1 -> Product2/1, Product1/2
  Divide/1 -> Add1/2
  Constant4/1 -> Add/2
  Product2/1 -> Divide2/2
  Constant5/1 -> Square/1
  Product/1 -> Square1/1
  Constant8/1 -> Product2/2
  Switch/1 -> Add1/3
  Constant/1 -> Switch/3
  Add/1 -> Gain/1
  Divide1/1 -> Switch/1
  Divide2/1 -> Add1/4
  Gain/1 -> Divide/1
  Square/1 -> Divide2/1, Divide1/1, Divide/2
  Square2/1 -> Product2/3
  Constant9/1 -> Square2/1
  Product1/1 -> Divide1/2
  In2/1 -> Product/2  "gear_ratio"
  Add1/1 -> Out1/1  "veh_eq_mass"
  data2/1 -> Switch/2  "ice_state"
  Constant2/1 -> Add1/1
  Constant6/1 -> Product1/1
  Constant7/1 -> Product/1

== system VehicleBackKin/Vehicle environment/Vehicle dynamics/Final drive power computation-ICE on/Road load power computation ==
  <veh_spd> : Inport
  <veh_acc> : Inport  Port=2
  <grade> : Inport  Port=3
  fd_spd : Inport  Port=4
  In5 : Inport  Port=5
  Add : Sum
  Add1 : Sum  Inputs=+++
  Add2 : Sum
  Bus Creator : BusCreator  Inputs=3
  Constant : Constant  Value=veh.F2
  Constant1 : Constant  Value=veh.F1
  Constant2 : Constant  Value=veh.F0
  Constant3 : Constant  Value=veh.mass
  Constant4 : Constant  Value=wh.radius
  Constant5 : Constant  Value=fd.ratio
  Divide : Product  Inputs=**/
  Product{,1..4} (5 alike) : Product
  Sin : Trigonometry
  Square : Math  Operator=square
  deg-->rad : Gain  Gain=pi/180
  g : Gain  Gain=9.81
  m/s-->km/h : Gain  Gain=3.6
  F_tot : Outport
  wires:
  <veh_spd>/1 -> m/s-->km/h/1
  <grade>/1 -> deg-->rad/1
  deg-->rad/1 -> Sin/1
  Constant1/1 -> Product2/2
  Sin/1 -> g/1
  m/s-->km/h/1 -> Product2/1, Square/1
  Constant2/1 -> Add/1
  Constant3/1 -> Product1/1
  g/1 -> Product1/2
  Product2/1 -> Add1/2
  Product1/1 -> Add/2
  Product3/1 -> Add1/1
  Add1/1 -> Add2/1  "F_res"
  Add/1 -> Add1/3
  <veh_acc>/1 -> Product/1
  In5/1 -> Product/2  "veh_eq_mass"
  Add2/1 -> Divide/1, Bus Creator/1  "F_tot_iceon"
  Product/1 -> Add2/2  "F_acc"
  Constant/1 -> Product3/2
  Square/1 -> Product3/1
  Constant4/1 -> Divide/2
  Constant5/1 -> Divide/3
  Divide/1 -> Bus Creator/2, Product4/1  "fd_trq_iceon"
  fd_spd/1 -> Product4/2  "fd_spd"
  Product4/1 -> Bus Creator/3  "fd_pwr_iceon"
  Bus Creator/1 -> F_tot/1
